simulink model "ABS_contDyn_model_SMC_FZL_NN"  (R2024b)
settings: Solver=VariableStepAuto  StartTime=0.0  StopTime=tf  MaxStep=1e-3  RelTol=1e-3  EnableMultiTasking=on
values from neighbouring files (symbols this model uses):
  dt = 1e-3    (= 0.001)    [mainABS_SMC_FZL_NN.m]
  hv = 0.5    [mainABS_SMC_FZL_NN.m]
  init_speed = 100    [mainABS_SMC_FZL_NN.m]
  lambda1_th = 0.02    [mainABS_SMC_FZL_NN.m]
  lambda2_th = 0.01    [mainABS_SMC_FZL_NN.m]
  omega_act = 70    [mainABS_SMC_FZL_NN.m]
  omega_LPF = 100    [mainABS_SMC_FZL_NN.m]
  rho = 0.97    [mainABS_SMC_FZL_NN.m]
  rho_off = 0.9    [mainABS_SMC_FZL_NN.m]
  rho_on = 1.01    [mainABS_SMC_FZL_NN.m]
  tau_delay = 10e-3    (= 0.01)    [mainABS_SMC_FZL_NN.m]
  Tb_dot_max = k    (= 5000)    [mainABS_SMC_FZL_NN.m]
  Tb_max = 1500    [mainABS_SMC_FZL_NN.m]
  v_on = -1    [mainABS_SMC_FZL_NN.m]
  v_stop = -1    [mainABS_SMC_FZL_NN.m]
undefined symbols (not defined in the file or in its folder): auxdata, rnn, smc
libraries: simulink x4, dspsigops x2, fuzblock x1
settings Model: Creator=luca  LastModifiedBy=victorfajemirokun
settings SolverCC: AlgebraicLoopSolver=TrustRegion
settings DataIOCC: LimitDataPoints=on  ReturnWorkspaceOutputs=off
settings OptimizationCC: ReuseModelBlockBuffer=off  LifeSpan=inf
settings DebuggingCC: UnconnectedInputMsg=warning  UnconnectedOutputMsg=warning  UnconnectedLineMsg=warning  AllowSymbolicDim=off  SFUnexpectedBacktrackingDiag=warning  SFNoUnconditionalDefaultTransitionDiag=warning  SFExecutionAtInitializationDiag=none  ArithmeticOperatorsInVariantConditions=warning
settings ModelReferenceCC: EnableRefExpFcnMdlSchedulingChecks=on  PropagateSignalLabelsOutOfModel=off
settings SFSimCC: SimUseLocalCustomCode=off  CustomCodeUndefinedFunction=UseInterfaceOnly
settings RTWCC: RTWUseLocalCustomCode=off  GPUComputeCapability=3.5
settings CodeAppCC: StateflowObjectComments=on
settings GRTTargetCC: TargetLangStandard=C89/C90 (ANSI)
settings ConfigComp: CovMetricSettings=dw  CovSaveCumulativeToWorkspaceVar=on  CovSaveSingleToWorkspaceVar=on  CovExternalEMLEnable=off

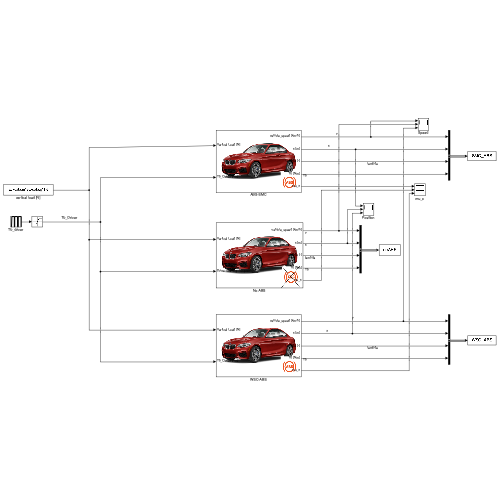
[thumbnail: Simulink's stored preview of the top-level diagram]
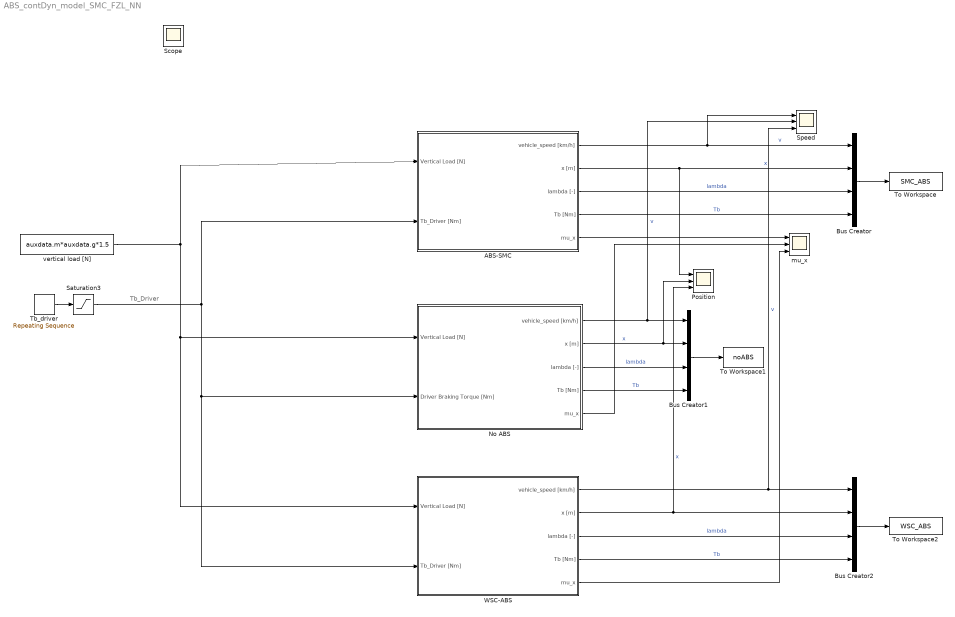
== system ABS_contDyn_model_SMC_FZL_NN ==
  note: Tb_Driver
  ABS-SMC : Subsystem
      mask Display: image('figures/ABScar_on.png');
  Bus Creator : BusCreator  Inputs=4
  Bus Creator1 : BusCreator  Inputs=4
  Bus Creator2 : BusCreator  Inputs=4
  No ABS : Subsystem
      mask Display: image('figures/ABS_off.png');
  Position : Scope  NumInputPorts=3
  Saturation3 : Saturate  UpperLimit=Tb_max  LowerLimit=0
  Speed : Scope  NumInputPorts=3
  Tb_driver : simulink/Sources/Repeating Sequence  rep_seq_t=time_manoeuvre  rep_seq_y=output_manoeuvre
  To Workspace : ToWorkspace  VariableName=SMC_ABS  SaveFormat=Timeseries  SampleTime=-1
  To Workspace1 : ToWorkspace  VariableName=noABS  SaveFormat=Timeseries  SampleTime=-1
  To Workspace2 : ToWorkspace  VariableName=WSC_ABS  SaveFormat=Timeseries  SampleTime=-1
  WSC-ABS : Subsystem
      mask Display: image('figures/ABScar_on.png');
  mu_x : Scope  NumInputPorts=3
  vertical load [N] : Constant  Value=auxdata.m*auxdata.g*1.5
  Scope : Scope
  wires:
  vertical load [N]/1 -> No ABS/1(Vertical Load [N]), WSC-ABS/1(Vertical Load [N]), ABS-SMC/1(Vertical Load [N])
  Saturation3/1 -> No ABS/2(Driver Braking Torque [Nm]), WSC-ABS/2(Tb_Driver [Nm]), ABS-SMC/2(Tb_Driver [Nm])
  No ABS/1(" vehicle_speed [km/h]") -> Speed/2, Bus Creator1/1  "v"
  No ABS/2(x [m]) -> Position/2, Bus Creator1/2  "x"
  ABS-SMC/1(vehicle_speed [km/h]) -> Bus Creator/1, Speed/1  "v"
  ABS-SMC/2(x [m]) -> Bus Creator/2, Position/1  "x"
  Bus Creator/1 -> To Workspace/1
  ABS-SMC/3(lambda [-]) -> Bus Creator/3  "lambda"
  ABS-SMC/4(Tb [Nm]) -> Bus Creator/4  "Tb"
  Bus Creator1/1 -> To Workspace1/1
  No ABS/3(lambda [-]) -> Bus Creator1/3  "lambda"
  No ABS/4(Tb [Nm]) -> Bus Creator1/4  "Tb"
  Tb_driver/1 -> Saturation3/1
  ABS-SMC/5(mu_x) -> mu_x/1
  No ABS/5(" mu_x") -> mu_x/2
  WSC-ABS/3(lambda [-]) -> Bus Creator2/3  "lambda"
  WSC-ABS/4(Tb [Nm]) -> Bus Creator2/4  "Tb"
  WSC-ABS/1(vehicle_speed [km/h]) -> Bus Creator2/1, Speed/3  "v"
  Bus Creator2/1 -> To Workspace2/1
  WSC-ABS/2(x [m]) -> Bus Creator2/2, Position/3  "x"
  WSC-ABS/5(mu_x) -> mu_x/3

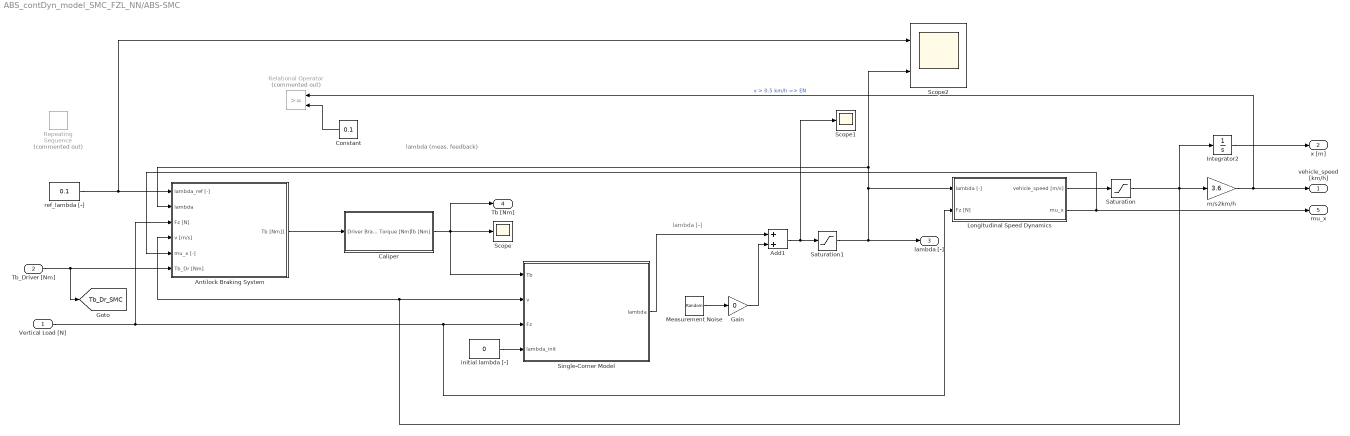
== system ABS_contDyn_model_SMC_FZL_NN/ABS-SMC ==
  note: lambda [-]
  note: lambda (meas. feedback)
  Vertical Load [N] : Inport
  Tb_Driver [Nm] : Inport  Port=2
  Add1 : Sum
  Antilock Braking System : Subsystem
      mask Display: image('figures/ABS_on.png');
  Caliper : Subsystem
  Constant : Constant  Value=0.1
  Gain : Gain  Gain=0
  Integrator2 : Integrator
  Longitudinal Speed Dynamics : Subsystem
  Measurement Noise : RandomNumber  Variance=2e-5  SampleTime=0.001
  Relational Operator : RelationalOperator  Commented=on  OutDataTypeStr=boolean  RndMeth=Simplest  InputSameDT=off
  Repeating Sequence : simulink/Sources/Repeating Sequence  Commented=on  rep_seq_t=time_manoeuvre  rep_seq_y=[0,0,0.1,0.1]
  Saturation : Saturate  UpperLimit=100  LowerLimit=1e-3
  Saturation1 : Saturate  UpperLimit=1  LowerLimit=0
  Scope : Scope
  Scope1 : Scope
  Scope2 : Scope  NumInputPorts=2
  Single-Corner Model : Subsystem
      mask Display:
      | image('figures/caliper_img.jpeg');
      | color('red');
      | port_label('output',1,'lambda');
      | port_label('input',1,'Tb');
      | port_label('input',2,'v');
      | port_label('input',3,'Fz');
      | port_label('input',4,'lambda_init');
  initial lambda [-] : Constant  Value=0
  m/s2km/h : Gain  Gain=3.6
  ref_lambda [-] : Constant  Value=0.1
  vehicle_speed [km/h] : Outport
  x [m] : Outport  Port=2
  lambda [-] : Outport  Port=3
  Tb [Nm] : Outport  Port=4
  mu_x : Outport  Port=5
  tag scope: Tb_Dr_SMC=global
  wires:
  m/s2km/h/1 -> Relational Operator/1, vehicle_speed [km/h]/1  "v > 0.5 km/h => EN"
  Integrator2/1 -> x [m]/1
  Longitudinal Speed Dynamics/1(vehicle_speed [m/s]) -> Saturation/1
  Caliper/1(Tb [Nm]) -> Single-Corner Model/1(Tb), Scope/1, Tb [Nm]/1
  Saturation1/1 -> Antilock Braking System/2(lambda), Scope2/2, Longitudinal Speed Dynamics/1(lambda [-]), lambda [-]/1
  Gain/1 -> Add1/2
  Tb_Driver [Nm]/1 -> [Tb_Dr_SMC], Antilock Braking System/6(Tb_Dr [Nm])
  Single-Corner Model/1(lambda) -> Add1/1
  Saturation/1 -> Single-Corner Model/2(v), Antilock Braking System/4(v [m/s]), Integrator2/1, m/s2km/h/1
  Add1/1 -> Saturation1/1, Scope1/1
  Measurement Noise/1 -> Gain/1
  initial lambda [-]/1 -> Single-Corner Model/4(lambda_init)
  Longitudinal Speed Dynamics/2(mu_x) -> Antilock Braking System/5(mu_x [-]), mu_x/1
  Vertical Load [N]/1 -> Antilock Braking System/3(Fz [N]), Single-Corner Model/3(Fz), Longitudinal Speed Dynamics/2(Fz [N])
  Constant/1 -> Relational Operator/2
  ref_lambda [-]/1 -> Antilock Braking System/1(lambda_ref [-]), Scope2/1
  Antilock Braking System/1(Tb [Nm]1) -> Caliper/1(Driver Braking Torque [Nm])

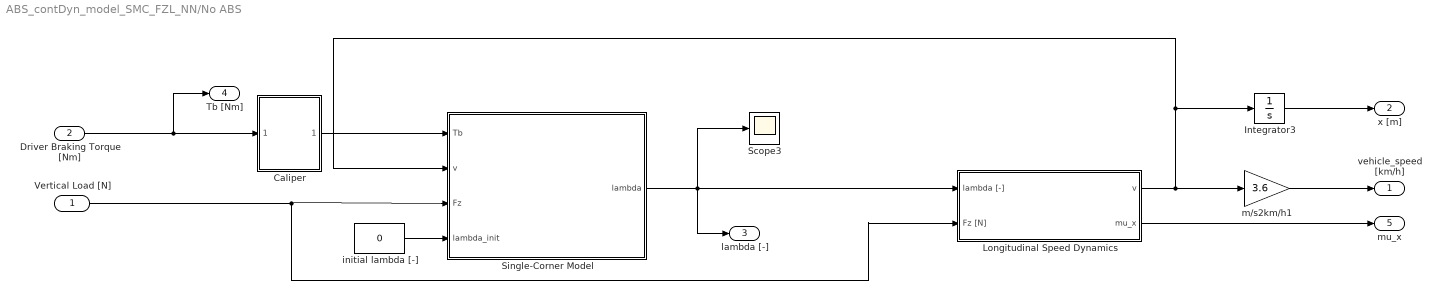
== system ABS_contDyn_model_SMC_FZL_NN/No ABS ==
  Vertical Load [N] : Inport
  Driver Braking Torque [Nm] : Inport  Port=2
  Caliper : Subsystem
  Integrator3 : Integrator
  Longitudinal Speed Dynamics : Subsystem
  Scope3 : Scope
  Single-Corner Model : Subsystem
      mask Display:
      | image('figures/caliper_img.jpeg');
      | color('red');
      | port_label('output',1,'lambda');
      | port_label('input',1,'Tb');
      | port_label('input',2,'v');
      | port_label('input',3,'Fz');
      | port_label('input',4,'lambda_init');
  initial lambda [-] : Constant  Value=0
  m/s2km/h1 : Gain  Gain=3.6
  " vehicle_speed [km/h]" : Outport
  x [m] : Outport  Port=2
  lambda [-] : Outport  Port=3
  Tb [Nm] : Outport  Port=4
  " mu_x" : Outport  Port=5
  wires:
  Single-Corner Model/1(lambda) -> lambda [-]/1, Longitudinal Speed Dynamics/1(lambda [-]), Scope3/1
  Vertical Load [N]/1 -> Longitudinal Speed Dynamics/2(Fz [N]), Single-Corner Model/3(Fz)
  Driver Braking Torque [Nm]/1 -> Tb [Nm]/1, Caliper/1(Driver Braking Torque [Nm])
  initial lambda [-]/1 -> Single-Corner Model/4(lambda_init)
  m/s2km/h1/1 -> " vehicle_speed [km/h]"/1
  Integrator3/1 -> x [m]/1
  Longitudinal Speed Dynamics/1(v) -> Integrator3/1, Single-Corner Model/2(v), m/s2km/h1/1
  Longitudinal Speed Dynamics/2(mu_x) -> " mu_x"/1
  Caliper/1(Tb [Nm]) -> Single-Corner Model/1(Tb)

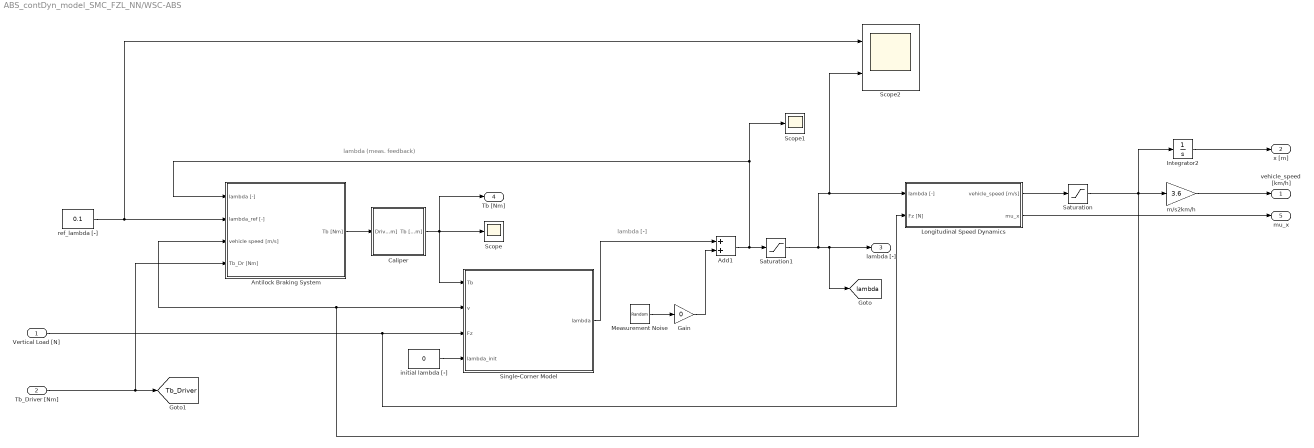
== system ABS_contDyn_model_SMC_FZL_NN/WSC-ABS ==
  note: lambda [-]
  note: lambda (meas. feedback)
  Vertical Load [N] : Inport
  Tb_Driver [Nm] : Inport  Port=2
  Add1 : Sum
  Antilock Braking System : Subsystem
      mask Display: image('figures/ABS_on.png');
  Caliper : Subsystem
  Gain : Gain  Gain=0
  Integrator2 : Integrator
  Longitudinal Speed Dynamics : Subsystem
  Measurement Noise : RandomNumber  Variance=2e-5  SampleTime=0.001
  Saturation : Saturate  UpperLimit=100  LowerLimit=1e-3
  Saturation1 : Saturate  UpperLimit=1  LowerLimit=0
  Scope : Scope
  Scope1 : Scope
  Scope2 : Scope  NumInputPorts=2
  Single-Corner Model : Subsystem
      mask Display:
      | image('figures/caliper_img.jpeg');
      | color('red');
      | port_label('output',1,'lambda');
      | port_label('input',1,'Tb');
      | port_label('input',2,'v');
      | port_label('input',3,'Fz');
      | port_label('input',4,'lambda_init');
  initial lambda [-] : Constant  Value=0
  m/s2km/h : Gain  Gain=3.6
  ref_lambda [-] : Constant  Value=0.1
  vehicle_speed [km/h] : Outport
  x [m] : Outport  Port=2
  lambda [-] : Outport  Port=3
  Tb [Nm] : Outport  Port=4
  mu_x : Outport  Port=5
  tag scope: Tb_Driver=global, lambda=global
  wires:
  m/s2km/h/1 -> vehicle_speed [km/h]/1
  Integrator2/1 -> x [m]/1
  Longitudinal Speed Dynamics/1(vehicle_speed [m/s]) -> Saturation/1
  Caliper/1(Tb [Nm]) -> Tb [Nm]/1, Single-Corner Model/1(Tb), Scope/1
  Saturation1/1 -> [lambda], lambda [-]/1, Scope2/2, Longitudinal Speed Dynamics/1(lambda [-])
  Gain/1 -> Add1/2
  Tb_Driver [Nm]/1 -> Antilock Braking System/4(Tb_Dr [Nm]), [Tb_Driver]
  Single-Corner Model/1(lambda) -> Add1/1
  Saturation/1 -> Single-Corner Model/2(v), Antilock Braking System/3(vehicle speed [m/s]), Integrator2/1, m/s2km/h/1
  Add1/1 -> Saturation1/1, Scope1/1, Antilock Braking System/1(lambda [-])
  Measurement Noise/1 -> Gain/1
  Vertical Load [N]/1 -> Single-Corner Model/3(Fz), Longitudinal Speed Dynamics/2(Fz [N])
  initial lambda [-]/1 -> Single-Corner Model/4(lambda_init)
  ref_lambda [-]/1 -> Scope2/1, Antilock Braking System/2(lambda_ref [-])
  Longitudinal Speed Dynamics/2(mu_x) -> mu_x/1
  Antilock Braking System/1(Tb [Nm]) -> Caliper/1(Driver Braking Torque [Nm])

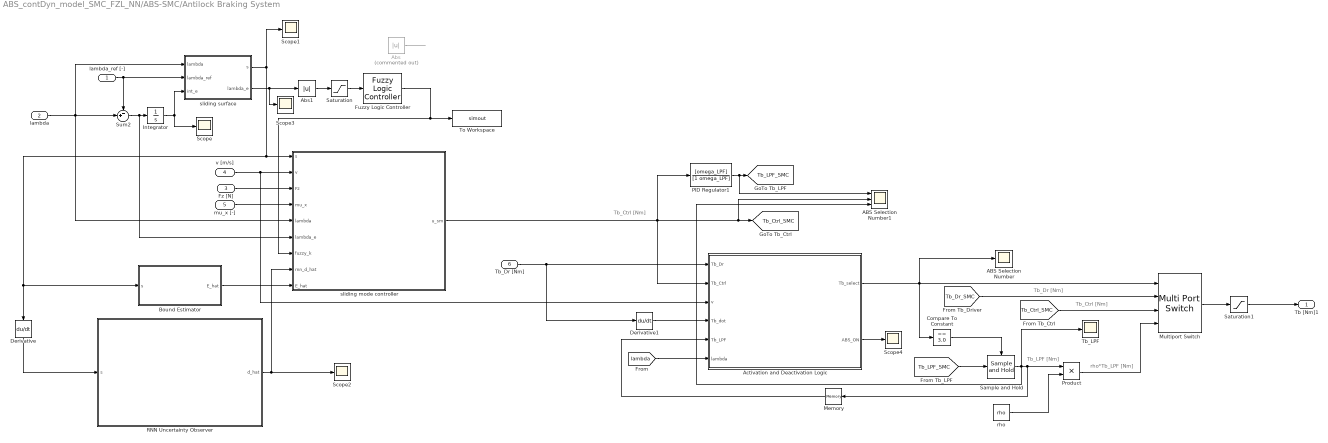
== system ABS_contDyn_model_SMC_FZL_NN/ABS-SMC/Antilock Braking System ==
  note: rho*Tb_LPF [Nm]
  note: Tb_Ctrl [Nm]
  note: Tb_Dr [Nm]
  note: Tb_Ctrl [Nm]
  note: Tb_LPF [Nm]
  lambda_ref [-] : Inport
  lambda : Inport  Port=2
  Fz [N] : Inport  Port=3
  v [m/s] : Inport  Port=4
  mu_x [-] : Inport  Port=5
  Tb_Dr [Nm] : Inport  Port=6
  ABS Selection Number : Scope
  ABS Selection Number1 : Scope  NumInputPorts=3
  Abs : Abs  Commented=on  SaturateOnIntegerOverflow=off
  Abs1 : Abs  SaturateOnIntegerOverflow=off
  Activation and Deactivation Logic : Stateflow chart  TreatAsAtomicUnit=on
  Bound Estimator : MATLAB Function  TreatAsAtomicUnit=on
  Compare To Constant : simulink/Logic and Bit Operations/Compare To Constant  relop===  const=3.0  OutDataTypeStr=boolean
  Derivative : Derivative
  Derivative1 : Derivative
  Fuzzy Logic Controller : fuzblock/Fuzzy Logic  Controller  FIS='fuzzy_smc.fis'  OutputSampleNumber=51  DataType=double  FuzzifiedInputs=off  RuleFiringStrengths=off  RuleOutputs=off  AggregatedOutputs=off  SimulateUsing=Interpreted execution  OutOfRangeInputValueMessage=warning  NoRuleFiredMessage=warning  EmptyOutputFuzzySetMessage=warning
  Integrator : Integrator
  Memory : Memory
  Multiport Switch : MultiPortSwitch  SaturateOnIntegerOverflow=off  InputSameDT=off
  PID Regulator1 : TransferFcn  Numerator=[omega_LPF]  Denominator=[1 omega_LPF]
  Product : Product
  RNN Uncertainty Observer : MATLAB Function  TreatAsAtomicUnit=on
  Sample and Hold : dspsigops/Sample and Hold  trig=Rising edge  initCond=0  latchinput=off
  Saturation : Saturate  UpperLimit=1  LowerLimit=0  LinearizeAsGain=off  ZeroCross=off
  Saturation1 : Saturate  UpperLimit=Tb_max  LowerLimit=0
  Scope{,1..4} (5 alike) : Scope
  Sum2 : Sum  Inputs=-+|
  Tb_LPF : Scope
  To Workspace : ToWorkspace  VariableName=simout  SaveFormat=Timeseries  SampleTime=-1
  rho : Constant  Value=rho
  sliding mode controller : MATLAB Function  TreatAsAtomicUnit=on
  sliding surface : MATLAB Function  TreatAsAtomicUnit=on
  Tb [Nm]1 : Outport
  tag scope: Tb_Ctrl_SMC=global, Tb_LPF_SMC=global
  wires:
  lambda/1 -> Sum2/2, sliding mode controller/5(lambda), sliding surface/1(lambda)
  lambda_ref [-]/1 -> Sum2/1, sliding surface/2(lambda_ref)
  Sum2/1 -> sliding mode controller/6(lambda_e), Integrator/1
  Integrator/1 -> Scope/1, sliding surface/3(int_e)
  mu_x [-]/1 -> sliding mode controller/4(mu_x)
  Fz [N]/1 -> sliding mode controller/3(Fz)
  Fuzzy Logic Controller/1 -> sliding mode controller/7(fuzzy_k), To Workspace/1
  Saturation/1 -> Fuzzy Logic Controller/1
  RNN Uncertainty Observer/1(d_hat) -> sliding mode controller/8(rnn_d_hat), Scope2/1
  Bound Estimator/1(E_hat) -> sliding mode controller/9(E_hat)
  sliding surface/1(s) -> Bound Estimator/1(s), Derivative/1, sliding mode controller/1(s), Scope1/1
  Derivative/1 -> RNN Uncertainty Observer/1(s)
  sliding surface/2(lambda_e) -> Abs1/1, Scope3/1
  Abs1/1 -> Saturation/1
  Saturation1/1 -> Tb [Nm]1/1
  Sample and Hold/1 -> Tb_LPF/1, ABS Selection Number1/3, Product/1, Memory/1
  sliding mode controller/1(u_sm) -> Activation and Deactivation Logic/2(Tb_Ctrl), [Tb_Ctrl_SMC], ABS Selection Number1/2, PID Regulator1/1
  [Tb_Ctrl_SMC] -> Multiport Switch/3
  [lambda] -> Activation and Deactivation Logic/6(lambda)
  Derivative1/1 -> Activation and Deactivation Logic/4(Tb_dot)
  Activation and Deactivation Logic/2(ABS_ON) -> Scope4/1
  Memory/1 -> Activation and Deactivation Logic/5(Tb_LPF)
  Tb_Dr [Nm]/1 -> Activation and Deactivation Logic/1(Tb_Dr), Derivative1/1
  Compare To Constant/1 -> Sample and Hold/Trigger
  PID Regulator1/1 -> ABS Selection Number1/1, [Tb_LPF_SMC]
  Product/1 -> Multiport Switch/4
  [Tb_Dr_SMC] -> Multiport Switch/2
  rho/1 -> Product/2
  [Tb_LPF_SMC] -> Sample and Hold/1
  Multiport Switch/1 -> Saturation1/1
  Activation and Deactivation Logic/1(Tb_select) -> ABS Selection Number/1, Multiport Switch/1, Compare To Constant/1
  v [m/s]/1 -> sliding mode controller/2(v), Activation and Deactivation Logic/3(v)
  Abs/1 -> ?

== system ABS_contDyn_model_SMC_FZL_NN/ABS-SMC/Caliper ==
  Driver Braking Torque [Nm] : Inport
  G_caliper : TransferFcn  Numerator=1  Denominator=[1/omega_act 1]
  Time delay caliper : TransportDelay  DelayTime=tau_delay
  Tb [Nm] : Outport
  wires:
  Time delay caliper/1 -> Tb [Nm]/1
  Driver Braking Torque [Nm]/1 -> G_caliper/1
  G_caliper/1 -> Time delay caliper/1

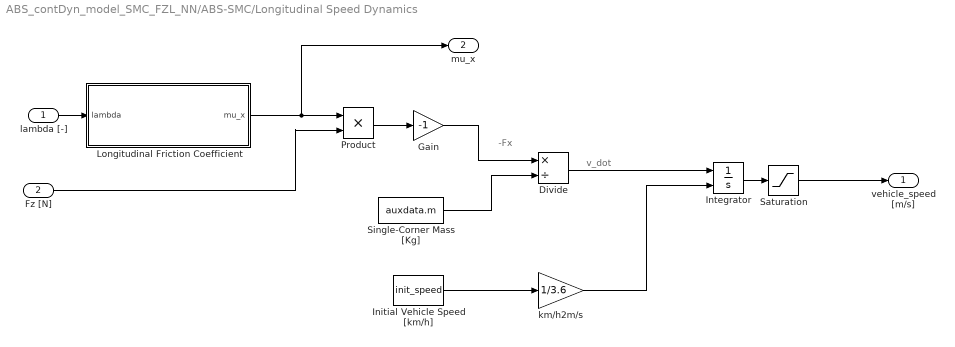
== system ABS_contDyn_model_SMC_FZL_NN/ABS-SMC/Longitudinal Speed Dynamics ==
  note: -Fx
  note: v_dot
  lambda [-] : Inport
  Fz [N] : Inport  Port=2
  Divide : Product  Inputs=*/
  Gain : Gain  Gain=-1
  Initial Vehicle Speed [km/h] : Constant  Value=init_speed
  Integrator : Integrator  InitialConditionSource=external
  Longitudinal Friction Coefficient : MATLAB Function  TreatAsAtomicUnit=on
  Product : Product
  Saturation : Saturate  UpperLimit=100  LowerLimit=0
  Single-Corner Mass [Kg] : Constant  Value=auxdata.m
  km/h2m/s : Gain  Gain=1/3.6
  vehicle_speed [m/s] : Outport
  mu_x : Outport  Port=2
  wires:
  Single-Corner Mass [Kg]/1 -> Divide/2
  Divide/1 -> Integrator/1
  km/h2m/s/1 -> Integrator/2
  Initial Vehicle Speed [km/h]/1 -> km/h2m/s/1
  Product/1 -> Gain/1
  Gain/1 -> Divide/1
  Saturation/1 -> vehicle_speed [m/s]/1
  Integrator/1 -> Saturation/1
  Longitudinal Friction Coefficient/1(mu_x) -> mu_x/1, Product/1
  Fz [N]/1 -> Product/2
  lambda [-]/1 -> Longitudinal Friction Coefficient/1(lambda)

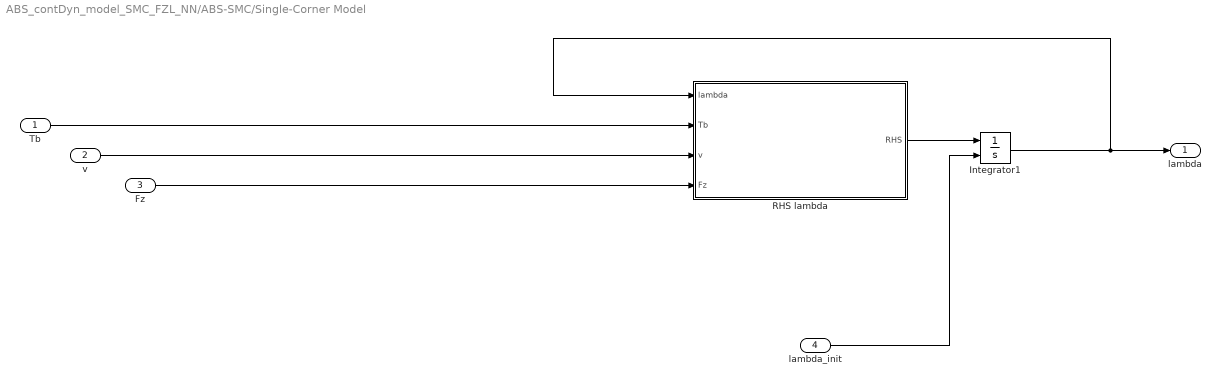
== system ABS_contDyn_model_SMC_FZL_NN/ABS-SMC/Single-Corner Model ==
  Tb : Inport
  v : Inport  Port=2
  Fz : Inport  Port=3
  lambda_init : Inport  Port=4
  Integrator1 : Integrator  InitialConditionSource=external  LimitOutput=on  UpperSaturationLimit=1  LowerSaturationLimit=0
  RHS lambda : MATLAB Function  TreatAsAtomicUnit=on
  lambda : Outport
  wires:
  lambda_init/1 -> Integrator1/2
  RHS lambda/1(RHS) -> Integrator1/1
  v/1 -> RHS lambda/3(v)
  Fz/1 -> RHS lambda/4(Fz)
  Integrator1/1 -> RHS lambda/1(lambda), lambda/1
  Tb/1 -> RHS lambda/2(Tb)

== system ABS_contDyn_model_SMC_FZL_NN/No ABS/Caliper ==
  Driver Braking Torque [Nm] : Inport
  G_caliper : TransferFcn  Numerator=1  Denominator=[1/omega_act 1]
  Time delay caliper : TransportDelay  DelayTime=tau_delay
  Tb [Nm] : Outport
  wires:
  Time delay caliper/1 -> Tb [Nm]/1
  Driver Braking Torque [Nm]/1 -> G_caliper/1
  G_caliper/1 -> Time delay caliper/1

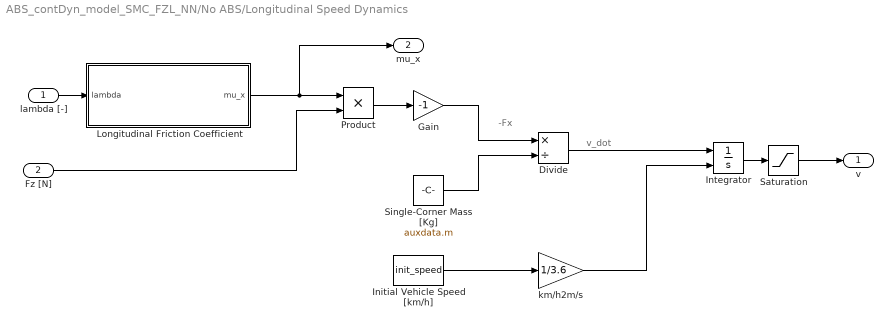
== system ABS_contDyn_model_SMC_FZL_NN/No ABS/Longitudinal Speed Dynamics ==
  note: -Fx
  note: v_dot
  lambda [-] : Inport
  Fz [N] : Inport  Port=2
  Divide : Product  Inputs=*/
  Gain : Gain  Gain=-1
  Initial Vehicle Speed [km/h] : Constant  Value=init_speed
  Integrator : Integrator  InitialConditionSource=external
  Longitudinal Friction Coefficient : MATLAB Function  TreatAsAtomicUnit=on
  Product : Product
  Saturation : Saturate  UpperLimit=100  LowerLimit=1e-3
  Single-Corner Mass [Kg] : Constant  Value=auxdata.m
  km/h2m/s : Gain  Gain=1/3.6
  v : Outport
  mu_x : Outport  Port=2
  wires:
  Single-Corner Mass [Kg]/1 -> Divide/2
  Divide/1 -> Integrator/1
  km/h2m/s/1 -> Integrator/2
  Initial Vehicle Speed [km/h]/1 -> km/h2m/s/1
  Product/1 -> Gain/1
  Gain/1 -> Divide/1
  Saturation/1 -> v/1
  Integrator/1 -> Saturation/1
  Longitudinal Friction Coefficient/1(mu_x) -> mu_x/1, Product/1
  Fz [N]/1 -> Product/2
  lambda [-]/1 -> Longitudinal Friction Coefficient/1(lambda)

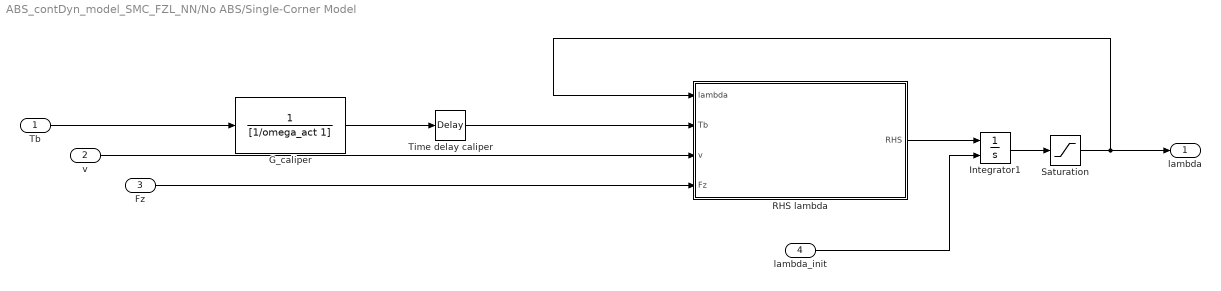
== system ABS_contDyn_model_SMC_FZL_NN/No ABS/Single-Corner Model ==
  Tb : Inport
  v : Inport  Port=2
  Fz : Inport  Port=3
  lambda_init : Inport  Port=4
  G_caliper : TransferFcn  Numerator=1  Denominator=[1/omega_act 1]
  Integrator1 : Integrator  InitialConditionSource=external
  RHS lambda : MATLAB Function  TreatAsAtomicUnit=on
  Saturation : Saturate  UpperLimit=0.99  LowerLimit=0
  Time delay caliper : TransportDelay  DelayTime=tau_delay
  lambda : Outport
  wires:
  lambda_init/1 -> Integrator1/2
  RHS lambda/1(RHS) -> Integrator1/1
  v/1 -> RHS lambda/3(v)
  Fz/1 -> RHS lambda/4(Fz)
  Integrator1/1 -> Saturation/1
  G_caliper/1 -> Time delay caliper/1
  Time delay caliper/1 -> RHS lambda/2(Tb)
  Tb/1 -> G_caliper/1
  Saturation/1 -> RHS lambda/1(lambda), lambda/1

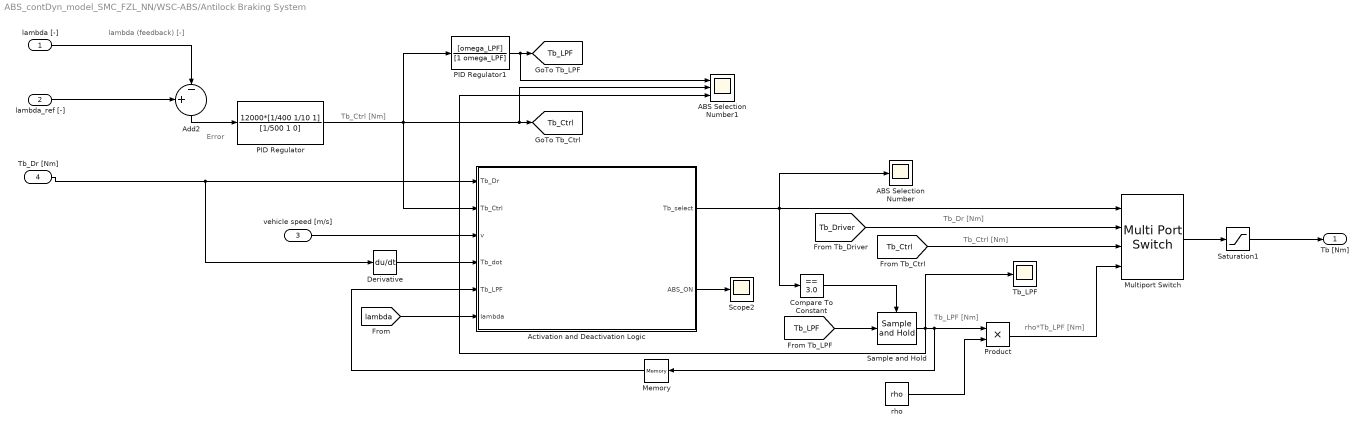
== system ABS_contDyn_model_SMC_FZL_NN/WSC-ABS/Antilock Braking System ==
  note: Tb_LPF [Nm]
  note: Tb_Ctrl [Nm]
  note: Tb_Dr [Nm]
  note: lambda (feedback) [-]
  note: Error
  note: Tb_Ctrl [Nm]
  note: rho*Tb_LPF [Nm]
  lambda [-] : Inport
  lambda_ref [-] : Inport  Port=2
  vehicle speed [m/s] : Inport  Port=3
  Tb_Dr [Nm] : Inport  Port=4
  ABS Selection Number : Scope
  ABS Selection Number1 : Scope  NumInputPorts=3
  Activation and Deactivation Logic : Stateflow chart  TreatAsAtomicUnit=on
  Add2 : Sum  Inputs=+-|
  Compare To Constant : simulink/Logic and Bit Operations/Compare To Constant  relop===  const=3.0  OutDataTypeStr=boolean
  Derivative : Derivative
  Memory : Memory
  Multiport Switch : MultiPortSwitch  SaturateOnIntegerOverflow=off  InputSameDT=off
  PID Regulator : TransferFcn  Numerator=12000*[1/400 1/10 1]  Denominator=[1/500 1 0]
  PID Regulator1 : TransferFcn  Numerator=[omega_LPF]  Denominator=[1 omega_LPF]
  Product : Product
  Sample and Hold : dspsigops/Sample and Hold  trig=Rising edge  initCond=0  latchinput=off
  Saturation1 : Saturate  UpperLimit=Tb_max  LowerLimit=0
  Scope2 : Scope
  Tb_LPF : Scope
  rho : Constant  Value=rho
  Tb [Nm] : Outport
  tag scope: Tb_Ctrl=global, Tb_LPF=global
  wires:
  lambda_ref [-]/1 -> Add2/1
  Activation and Deactivation Logic/2(ABS_ON) -> Scope2/1
  [Tb_Ctrl] -> Multiport Switch/3
  lambda [-]/1 -> Add2/2
  Tb_Dr [Nm]/1 -> Derivative/1, Activation and Deactivation Logic/1(Tb_Dr)
  vehicle speed [m/s]/1 -> Activation and Deactivation Logic/3(v)
  Multiport Switch/1 -> Saturation1/1
  Add2/1 -> PID Regulator/1
  [Tb_Driver] -> Multiport Switch/2
  Derivative/1 -> Activation and Deactivation Logic/4(Tb_dot)
  [lambda] -> Activation and Deactivation Logic/6(lambda)
  Activation and Deactivation Logic/1(Tb_select) -> ABS Selection Number/1, Multiport Switch/1, Compare To Constant/1
  Saturation1/1 -> Tb [Nm]/1
  PID Regulator/1 -> PID Regulator1/1, ABS Selection Number1/2, [Tb_Ctrl], Activation and Deactivation Logic/2(Tb_Ctrl)
  PID Regulator1/1 -> ABS Selection Number1/1, [Tb_LPF]
  Compare To Constant/1 -> Sample and Hold/Trigger
  [Tb_LPF] -> Sample and Hold/1
  Sample and Hold/1 -> Tb_LPF/1, ABS Selection Number1/3, Product/1, Memory/1
  Memory/1 -> Activation and Deactivation Logic/5(Tb_LPF)
  rho/1 -> Product/2
  Product/1 -> Multiport Switch/4

== system ABS_contDyn_model_SMC_FZL_NN/WSC-ABS/Caliper ==
  Driver Braking Torque [Nm] : Inport
  G_caliper : TransferFcn  Numerator=1  Denominator=[1/omega_act 1]
  Time delay caliper : TransportDelay  DelayTime=tau_delay
  Tb [Nm] : Outport
  wires:
  Time delay caliper/1 -> Tb [Nm]/1
  Driver Braking Torque [Nm]/1 -> G_caliper/1
  G_caliper/1 -> Time delay caliper/1

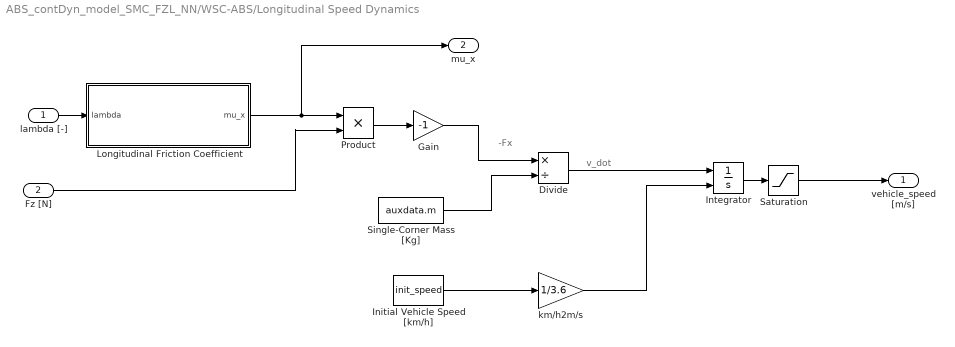
== system ABS_contDyn_model_SMC_FZL_NN/WSC-ABS/Longitudinal Speed Dynamics ==
  note: -Fx
  note: v_dot
  lambda [-] : Inport
  Fz [N] : Inport  Port=2
  Divide : Product  Inputs=*/
  Gain : Gain  Gain=-1
  Initial Vehicle Speed [km/h] : Constant  Value=init_speed
  Integrator : Integrator  InitialConditionSource=external
  Longitudinal Friction Coefficient : MATLAB Function  TreatAsAtomicUnit=on
  Product : Product
  Saturation : Saturate  UpperLimit=100  LowerLimit=0
  Single-Corner Mass [Kg] : Constant  Value=auxdata.m
  km/h2m/s : Gain  Gain=1/3.6
  vehicle_speed [m/s] : Outport
  mu_x : Outport  Port=2
  wires:
  Single-Corner Mass [Kg]/1 -> Divide/2
  Divide/1 -> Integrator/1
  km/h2m/s/1 -> Integrator/2
  Initial Vehicle Speed [km/h]/1 -> km/h2m/s/1
  Product/1 -> Gain/1
  Gain/1 -> Divide/1
  Saturation/1 -> vehicle_speed [m/s]/1
  Integrator/1 -> Saturation/1
  Longitudinal Friction Coefficient/1(mu_x) -> mu_x/1, Product/1
  Fz [N]/1 -> Product/2
  lambda [-]/1 -> Longitudinal Friction Coefficient/1(lambda)

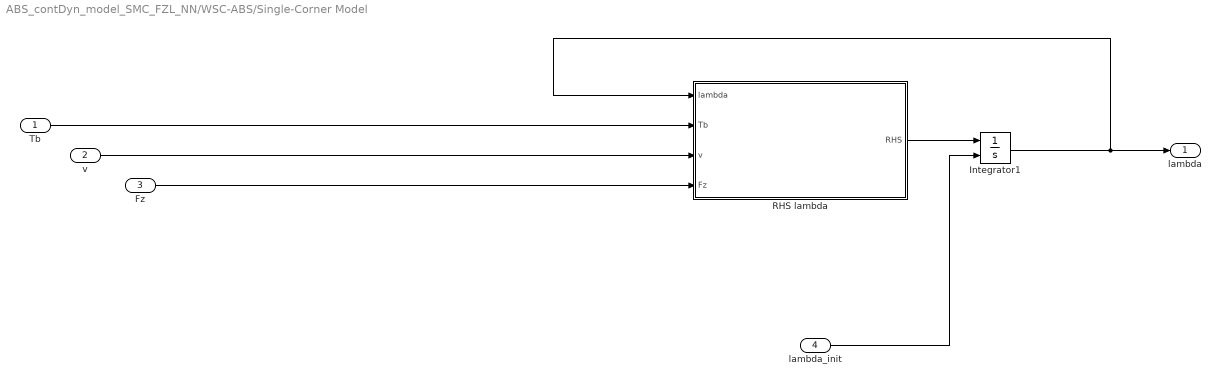
== system ABS_contDyn_model_SMC_FZL_NN/WSC-ABS/Single-Corner Model ==
  Tb : Inport
  v : Inport  Port=2
  Fz : Inport  Port=3
  lambda_init : Inport  Port=4
  Integrator1 : Integrator  InitialConditionSource=external  LimitOutput=on  UpperSaturationLimit=1  LowerSaturationLimit=0
  RHS lambda : MATLAB Function  TreatAsAtomicUnit=on
  lambda : Outport
  wires:
  lambda_init/1 -> Integrator1/2
  RHS lambda/1(RHS) -> Integrator1/1
  v/1 -> RHS lambda/3(v)
  Fz/1 -> RHS lambda/4(Fz)
  Integrator1/1 -> RHS lambda/1(lambda), lambda/1
  Tb/1 -> RHS lambda/2(Tb)

== matlab function ABS_contDyn_model_SMC_FZL_NN/ABS-SMC/Antilock Braking System/sliding surface ==
  data: lambda input; s output; lambda_ref input; int_e input; smc parameter; lambda_e output
function [s, lambda_e] = ss(lambda, lambda_ref, int_e, smc)

    lambda_e = lambda - lambda_ref;
    s = lambda_e + smc.k*int_e;

== matlab function ABS_contDyn_model_SMC_FZL_NN/ABS-SMC/Single-Corner Model/RHS lambda ==
  data: lambda input; RHS output; Tb input; v input; Fz input; auxdata parameter
function RHS = lambdaDyn( lambda, Tb, v, Fz, auxdata )
% Right hand side of the longitudinal slip dynamics

omega = (1 - lambda) * v / auxdata.r_w;

% Equilibrium manifold
%        /      (1 - lambda) * J \
% Psi = | r_w + ----------------  | * Fz * mu
%        \          r_w * m      /
Psi = (auxdata.r_w + ...
       auxdata.J / (auxdata.r_w * auxdata.m) * (1 - lambda)) * Fz * ...
       burckhardt( lambda, auxdata.road_condition );


if omega <= 0.1
    RHS = 0;
else
    RHS = -(1 - lambda) / (auxdata.J * omega) * (Psi - Tb);
end

end

== matlab function ABS_contDyn_model_SMC_FZL_NN/WSC-ABS/Single-Corner Model/RHS lambda ==
  data: lambda input; RHS output; Tb input; v input; Fz input; auxdata parameter
function RHS = lambdaDyn( lambda, Tb, v, Fz, auxdata )
% Right hand side of the longitudinal slip dynamics

omega = (1 - lambda) * v / auxdata.r_w;

% Equilibrium manifold
%        /      (1 - lambda) * J \
% Psi = | r_w + ----------------  | * Fz * mu
%        \          r_w * m      /
Psi = (auxdata.r_w + ...
       auxdata.J / (auxdata.r_w * auxdata.m) * (1 - lambda)) * Fz * ...
       burckhardt( lambda, auxdata.road_condition );


if omega <= 0.1
    RHS = 0;
else
    RHS = -(1 - lambda) / (auxdata.J * omega) * (Psi - Tb);
end

end

== matlab function ABS_contDyn_model_SMC_FZL_NN/ABS-SMC/Antilock Braking System/sliding mode controller ==
  data: s input; v input; Fz input; mu_x input; lambda input; lambda_e input; u_sm output; auxdata parameter; smc parameter; fuzzy_k input; rnn_d_hat input; E_hat input
function u_sm = smc(s, v, Fz, mu_x, lambda, lambda_e, auxdata, smc, fuzzy_k, rnn_d_hat, E_hat)

    % compute nominal drift f_n and control gain g_n
    fn = -(1/v)*(((1 - lambda)/auxdata.m) + auxdata.r_w^2/auxdata.J) * Fz * mu_x;
    gn =  (  auxdata.r_w   )/(auxdata.J * v);

    lambda_ref_dot = 0;

    % Equivalent controller
    u_eq = (-fn + lambda_ref_dot - smc.k*lambda_e - rnn_d_hat) / gn;
    % u_eq = (-fn + lambda_ref_dot - fuzzy_k*lambda_e - rnn_d_hat) / gn;

    % robust controller
    % u_r = -smc.rho*sign(s) / gn;
    u_r = - E_hat * sign(s) / gn;
    
    % smc control command
    u_sm = u_eq + u_r;
end

== matlab function ABS_contDyn_model_SMC_FZL_NN/ABS-SMC/Antilock Braking System/Bound Estimator ==
  settings: updateMethod=DISCRETE  sampleTime=dt
  data: s input; E_hat output; rnn parameter; dt parameter
function E_hat = bound_estimator(s, rnn, dt)

    persistent init_flag E_hat_pers;

    if (isempty(init_flag))
        E_hat_pers = 0;

        init_flag = 1;
    end

    epsilon = 0.05;

    E_hat_dot = rnn.eta5 * (abs(s) - epsilon*E_hat_pers);
    % E_hat_dot = rnn.eta5 * abs(s);
    E_hat_pers =   E_hat_pers + E_hat_dot*dt;

    E_hat = max(E_hat_pers, 0);
end

== matlab function ABS_contDyn_model_SMC_FZL_NN/ABS-SMC/Antilock Braking System/RNN Uncertainty Observer ==
  settings: updateMethod=DISCRETE
  data: s input; d_hat output; rnn parameter; dt parameter
function d_hat = rnn_uncertainty_observer(s, rnn, dt)
    
    % static initialization flag
    persistent init_flag;
    % static variables of the rnn parameters updated ONLINE
    persistent alpha_hat v_hat w_hat r_hat Theta_hat;

    if (isempty(init_flag))
        rng("shuffle"); % seed random number generator
        % initialize to gaussian/normal random small weights
        alpha_hat = 0.01 * randn(rnn.neuron_N, 1); % weights between hidden layer and output layer

        % initialize center of RBF to range of input (s, i.e lambda_e)
        % v_hat = transpose(linspace(-0.5, 0.5, rnn.neuron_N)); % center of radial basis function (RBF)
        v_hat = normrnd(0,0.05, [rnn.neuron_N, 1]);
        
        % initialize RBF width to small random values according
        % gaussian/normal distribution
        % w_hat = 0.1 * rand(rnn.neuron_N, 1) + 2; % inverse of width (spread i.e. 1/sigma^2) of radial basis function (RBF)
        w_hat = normrnd(2, 0.1, [rnn.neuron_N, 1]); % inverse of width (spread i.e. 1/sigma^2) of radial basis function (RBF)

        % initialize recurrent 
        r_hat = 0.1 * randn(rnn.neuron_N, 1); % internal feedback gain

        Theta_hat = zeros(rnn.neuron_N, 1); % firing weight of the k-th neuron in the hidden layer

        init_flag = 1;
    end

    % Initialise derivatives matrices
    A = zeros(rnn.neuron_N, rnn.neuron_N);
    B = zeros(rnn.neuron_N, rnn.neuron_N);
    C = zeros(rnn.neuron_N, rnn.neuron_N);

    theta_last = Theta_hat;

    for k = 1:rnn.neuron_N
        dnetk_dv = -2 * w_hat(k)^2 * (s + theta_last(k)*r_hat(k) - v_hat(k));
        dnetk_dw = 2 * w_hat(k) * (s + theta_last(k)*r_hat(k) - v_hat(k))^2;
        dnetk_dr = 2 * theta_last(k) * w_hat(k)^2 * (s + theta_last(k)*r_hat(k) - v_hat(k));

        net_k = w_hat(k)^2 * (s + Theta_hat(k)*r_hat(k) - v_hat(k))^2;
        Theta_hat(k) = exp(-net_k);

        A(k,k) = -Theta_hat(k) * dnetk_dv;
        B(k,k) = -Theta_hat(k) * dnetk_dw;
        C(k,k) = -Theta_hat(k) * dnetk_dr;
    end

    d_hat = transpose(alpha_hat) * Theta_hat;

    alpha_hat_dot = rnn.eta1 * s * Theta_hat;
    v_hat_dot = rnn.eta2 * s * A * alpha_hat;
    w_hat_dot = rnn.eta3 * s * B * alpha_hat;
    r_hat_dot = rnn.eta4 * s * C * alpha_hat;

    alpha_hat = alpha_hat + alpha_hat_dot*dt;
    v_hat = v_hat + v_hat_dot*dt;
    w_hat = w_hat + w_hat_dot*dt;
    r_hat = r_hat + r_hat_dot*dt;
    % alpha_hat = alpha_hat + alpha_hat_dot;
    % v_hat = v_hat + v_hat_dot;
    % w_hat = w_hat + w_hat_dot;
    % r_hat = r_hat + r_hat_dot;
end

== stateflow chart ABS_contDyn_model_SMC_FZL_NN/ABS-SMC/Antilock Braking System/Activation and Deactivation Logic ==
  state High_Speed_ON
    entry: Tb_select = 2;
    entry: ABS_ON = true;
  state High_Speed_OFF
    entry: Tb_select = 1;
    entry: ABS_ON = false;
  state Low_Speed_ON
    entry: Tb_select = 3;
    entry: ABS_ON = true;
  state Low_Speed_OFF
    entry: Tb_select = 1;
    entry: ABS_ON = false;
  High_Speed_OFF -> High_Speed_ON [order 1] : [lambda > lambda1_th - (lambda1_th - lambda2_th)/Tb_dot_max*Tb_dot && ...
      |  Tb_Dr > rho_on*Tb_Ctrl && ...
      |  v > v_on]
  (default) -> High_Speed_OFF : {Tb_select = 1;}
  High_Speed_ON -> High_Speed_OFF [order 1] : [Tb_Dr < rho_off*Tb_Ctrl]
  High_Speed_OFF -> Low_Speed_OFF [order 2] : [v < v_on -hv]
  Low_Speed_OFF -> High_Speed_OFF : [v > v_on +hv]
  High_Speed_ON -> Low_Speed_ON [order 2] : [v < v_on]
  Low_Speed_ON -> Low_Speed_OFF : [v < v_stop || Tb_Dr < rho_off*Tb_LPF]
  data: Tb_select output; Tb_Dr input; Tb_Ctrl input; v input; Tb_dot input; Tb_dot_max parameter; v_on parameter; rho_on parameter; Tb_LPF input; lambda input; lambda1_th parameter; v_stop parameter; hv parameter; rho_off parameter; ABS_ON output; lambda2_th parameter

== stateflow chart ABS_contDyn_model_SMC_FZL_NN/WSC-ABS/Antilock Braking System/Activation and Deactivation Logic ==
  state High_Speed_ON
    entry: Tb_select = 2;
    entry: ABS_ON = true;
  state High_Speed_OFF
    entry: Tb_select = 1;
    entry: ABS_ON = false;
  state Low_Speed_ON
    entry: Tb_select = 3;
    entry: ABS_ON = true;
  state Low_Speed_OFF
    entry: Tb_select = 1;
    entry: ABS_ON = false;
  High_Speed_OFF -> High_Speed_ON [order 1] : [lambda > lambda1_th - (lambda1_th - lambda2_th)/Tb_dot_max*Tb_dot && ...
      |  Tb_Dr > rho_on*Tb_Ctrl && ...
      |  v > v_on]
  (default) -> High_Speed_OFF : {Tb_select = 1;}
  High_Speed_ON -> High_Speed_OFF [order 1] : [Tb_Dr < rho_off*Tb_Ctrl]
  High_Speed_OFF -> Low_Speed_OFF [order 2] : [v < v_on -hv]
  Low_Speed_OFF -> High_Speed_OFF : [v > v_on +hv]
  High_Speed_ON -> Low_Speed_ON [order 2] : [v < v_on]
  Low_Speed_ON -> Low_Speed_OFF : [v < v_stop || Tb_Dr < rho_off*Tb_LPF]
  data: Tb_select output; Tb_Dr input; Tb_Ctrl input; v input; Tb_dot input; Tb_dot_max parameter; v_on parameter; rho_on parameter; Tb_LPF input; lambda input; lambda1_th parameter; v_stop parameter; hv parameter; rho_off parameter; ABS_ON output; lambda2_th parameter

== matlab function ABS_contDyn_model_SMC_FZL_NN/ABS-SMC/Longitudinal Speed Dynamics/Longitudinal Friction Coefficient ==
  data: lambda input; mu_x output; auxdata parameter
function mu_x = LongitudinalFrction(lambda,auxdata)
    
mu_x = burckhardt(lambda,auxdata.road_condition);

end

== matlab function ABS_contDyn_model_SMC_FZL_NN/No ABS/Single-Corner Model/RHS lambda ==
  data: lambda input; RHS output; Tb input; v input; Fz input; auxdata parameter
function RHS = lambdaDyn( lambda, Tb, v, Fz, auxdata )
% Right hand side of the longitudinal slip dynamics

omega = (1 - lambda) * v / auxdata.r_w;

% Equilibrium manifold
%        /      (1 - lambda) * J \
% Psi = | r_w + ----------------  | * Fz * mu
%        \          r_w * m      /
Psi = (auxdata.r_w + ...
       auxdata.J / (auxdata.r_w * auxdata.m) * (1 - lambda)) * Fz * ...
       burckhardt( lambda, auxdata.road_condition );

if omega <= 0.1
    RHS = 0;
else
    RHS = -(1 - lambda) / (auxdata.J * omega) * (Psi - Tb);
end

end

== matlab function ABS_contDyn_model_SMC_FZL_NN/WSC-ABS/Longitudinal Speed Dynamics/Longitudinal Friction Coefficient ==
  data: lambda input; mu_x output; auxdata parameter
function mu_x = LongitudinalFrction(lambda,auxdata)
    
mu_x = burckhardt(lambda,auxdata.road_condition);

end

== matlab function ABS_contDyn_model_SMC_FZL_NN/No ABS/Longitudinal Speed Dynamics/Longitudinal Friction Coefficient ==
  data: lambda input; mu_x output; auxdata parameter
function mu_x = LongitudinalFrction( lambda, auxdata )
    
mu_x = burckhardt( lambda, auxdata.road_condition );

end
